simulink model "fuelsys_htmreq"  (Simulink 6.0)
settings: Solver=ode3  SolverMode=SingleTasking  StartTime=0.0  StopTime=2000  FixedStep=0.001  RelTol=1e-5  AbsTol=1e-6
PreLoadFcn:
  | load fsysdat
undefined symbols (not defined in the file): A1, A2, B1, B2, DISABLED, DiscIntNeverNeededParam, hys, Ki, LOW, max_ego, max_press, max_speed, max_throt, min_press, min_throt, o2_t_thresh, PressEst, pumpCon, RICH, SpeedEst, ThrotEst, zero_thresh
libraries: simulink x5, simulink_extras x3
settings Model: CovMetricSettings=dcmtr  Creator=The MathWorks Inc.  LastModifiedBy=batserve  ExtModeTrigMode=oneshot  ExtModeArmWhenConnect=off  ExtModeAutoUpdateStatusClock=off
settings DataIOCC: LimitDataPoints=off  SaveOutput=off  SaveTime=off  SignalLoggingName=logsOut
settings OptimizationCC: OptimizeModelRefInitCode=on  LifeSpan=1
settings DebuggingCC: CheckExecutionContextPreStartOutputMsg=on  CheckExecutionContextRuntimeOutputMsg=on  SolverPrmCheckMsg=none  IntegerOverflowMsg=none
settings ModelReferenceCC: UpdateModelReferenceTargets=IfOutOfDate
settings RTWCC: SystemTargetFile=ert.tlc  TemplateMakefile=ert_default_tmf  Description=RTW Embedded Coder (no auto configuration)  ProcessScript=ert_make_rtw_hook
settings ERTTargetCC: TargetFcnLib=ansi_tfl_tmw.mat  GenFloatMathFcnCalls=ANSI_C  GenerateSampleERTMain=on  SupportContinuousTime=on  SupportNonInlinedSFcns=on  RootIOFormat=Individual Arguments  ERTCustomFileTemplate=example_file_process.tlc  InitialValueSource=Model

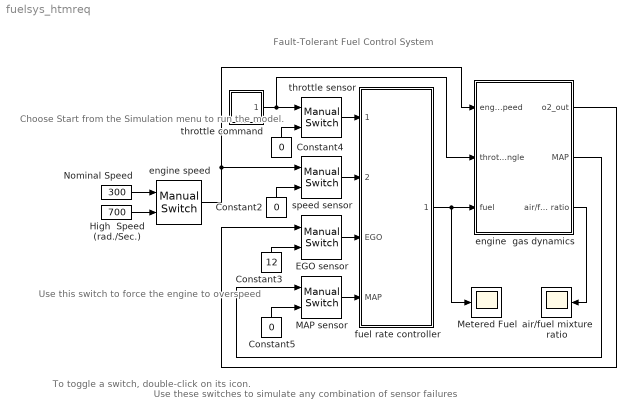
== system fuelsys_htmreq ==
  note: Use these switches to
      | simulate any combination
      | of sensor failures
  note: Use this switch
      | to force the
      | engine to
      | overspeed
  note: Fault-Tolerant Fuel Control System
  note: Choose Start from
      | the Simulation
      | menu to run
      | the model.
  note: To toggle
      | a switch,
      | double-click
      | on its icon.
  Constant2 : Constant  Orientation=up  Value=0
  Constant3 : Constant  Orientation=up  Value=12
  Constant4 : Constant  Orientation=up  Value=0
  Constant5 : Constant  Orientation=up  Value=0
  EGO sensor : simulink/Signal Routing/Manual Switch  sw=1  action=0
  High  Speed (rad./Sec.) : Constant  Value=700
  MAP sensor : simulink/Signal Routing/Manual Switch  sw=1  action=0
  Metered Fuel : Scope
      settings: TickLabels=on  TimeRange=8  YMin=0.75  YMax=2.25  DataFormat=Array
  Nominal Speed : Constant  Value=300
  air/fuel mixture ratio : Scope
      settings: TickLabels=on  TimeRange=8  YMin=11  YMax=16  DataFormat=Array
  engine speed : simulink/Signal Routing/Manual Switch  sw=1  action=0
  engine  gas dynamics : Subsystem  PropExecContextAcrossSSBoundary=on
  fuel rate controller : Subsystem  PropExecContextAcrossSSBoundary=on
  speed sensor : simulink/Signal Routing/Manual Switch  sw=1  action=0
  throttle command : Subsystem  PropExecContextAcrossSSBoundary=on  mask(Repeating table){rep_seq_t=[0 2 4], rep_seq_y=[10 20 10]}
      mask prompts: rep_seq_t "Time values:"; rep_seq_y "Output values:"
      mask help: Repeating table.
      mask init:
      | period = max(rep_seq_t);
      mask Help: Repeats cycle given in table. Time values should be monotonically increasing.
      mask Display: plot([rep_seq_t,rep_seq_t+period,rep_seq_t+2*period,rep_seq_t(1)+3*period],[rep_seq_y,rep_seq_y,rep_seq_y,rep_seq_y(1)])
  throttle sensor : simulink/Signal Routing/Manual Switch  sw=1  action=0
  wires:
  engine  gas dynamics/3(air/fuel ratio) -> air/fuel mixture ratio/1
  engine speed/1 -> engine  gas dynamics/1(engine speed), speed sensor/1
  MAP sensor/1 -> fuel rate controller/4(MAP)
  EGO sensor/1 -> fuel rate controller/3(EGO)
  speed sensor/1 -> fuel rate controller/2(engine speed)
  throttle sensor/1 -> fuel rate controller/1(throttle)
  fuel rate controller/1(fuel rate) -> engine  gas dynamics/3(fuel), Metered Fuel/1
  engine  gas dynamics/1(o2_out) -> EGO sensor/1
  Constant5/1 -> MAP sensor/2
  Constant3/1 -> EGO sensor/2
  throttle command/1(out_1) -> engine  gas dynamics/2(throttle angle), throttle sensor/1
  Constant2/1 -> speed sensor/2
  Constant4/1 -> throttle sensor/2
  engine  gas dynamics/2(MAP) -> MAP sensor/1
  High  Speed (rad./Sec.)/1 -> engine speed/2
  Nominal Speed/1 -> engine speed/1

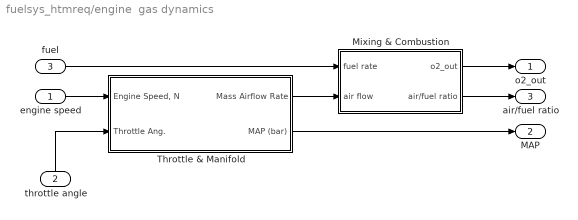
== system fuelsys_htmreq/engine  gas dynamics ==
  engine speed : Inport  Port=1  LatchInput=off
  throttle angle : Inport  Orientation=up  Port=2  LatchInput=off
  fuel : Inport  Port=3  LatchInput=off
  Mixing & Combustion : Subsystem  PropExecContextAcrossSSBoundary=on
  Throttle & Manifold : Subsystem  PropExecContextAcrossSSBoundary=on
  o2_out : Outport  InitialOutput=0
  MAP : Outport  Port=2  InitialOutput=0
  air/fuel ratio : Outport  Port=3  InitialOutput=0
  wires:
  Throttle & Manifold/1(Mass Airflow Rate) -> Mixing & Combustion/2(air flow)
  fuel/1 -> Mixing & Combustion/1(fuel rate)
  engine speed/1 -> Throttle & Manifold/1("Engine Speed, N")
  throttle angle/1 -> Throttle & Manifold/2(Throttle Ang.)
  Mixing & Combustion/2(air/fuel ratio) -> air/fuel ratio/1
  Throttle & Manifold/2(MAP (bar)) -> MAP/1
  Mixing & Combustion/1(o2_out) -> o2_out/1

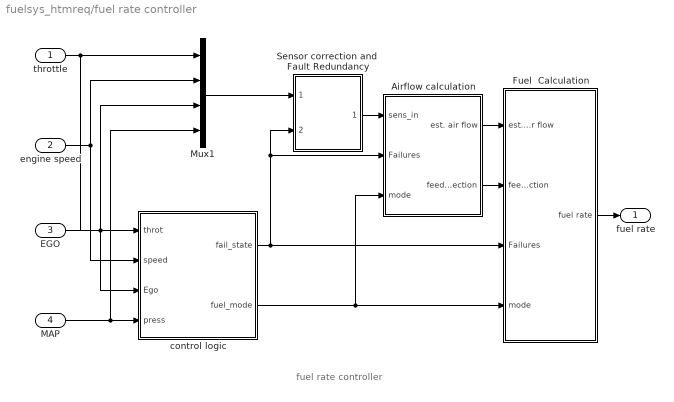
== system fuelsys_htmreq/fuel rate controller ==
  note: fuel rate controller
  throttle : Inport  Port=1  LatchInput=off
  engine speed : Inport  Port=2  LatchInput=off
  EGO : Inport  Port=3  LatchInput=off
  MAP : Inport  Port=4  LatchInput=off
  Airflow calculation : Subsystem  RequirementInfo={ 'HTML' 'fuelsys_requirements.htm' 'REQ1' 'true' 'Using a few parameters to estimate the mass airflow through the engine' 'REQ1' }  PropExecContextAcrossSSBoundary=on
  Fuel  Calculation : Subsystem  PropExecContextAcrossSSBoundary=on
  Mux1 : Mux
  Sensor correction and  Fault Redundancy : Subsystem  PropExecContextAcrossSSBoundary=on
  control logic : Stateflow chart  Description=Stateflow diagram to determine control system operating mode  PropExecContextAcrossSSBoundary=on
  fuel rate : Outport  InitialOutput=0
  wires:
  MAP/1 -> Mux1/4, control logic/4(press)
  EGO/1 -> Mux1/3, control logic/3(Ego)
  engine speed/1 -> Mux1/2, control logic/2(speed)
  throttle/1 -> Mux1/1, control logic/1(throt)
  Mux1/1 -> Sensor correction and  Fault Redundancy/1(Sensors)
  control logic/2(fuel_mode) -> Fuel  Calculation/4(mode), Airflow calculation/3(mode)
  Airflow calculation/2(feedback correction) -> Fuel  Calculation/2(feedback correction)
  Fuel  Calculation/1(fuel rate) -> fuel rate/1
  Airflow calculation/1(est. air flow) -> Fuel  Calculation/1(est. air flow)
  Sensor correction and  Fault Redundancy/1(Corrected) -> Airflow calculation/1(sens_in)
  control logic/1(fail_state) -> Sensor correction and  Fault Redundancy/2(Failures), Airflow calculation/2(Failures), Fuel  Calculation/3(Failures)

== system fuelsys_htmreq/throttle command ==
  Clock : Clock
      settings: Decimation=10
  Fcn1 : Fcn  Expr=rem(u[1],period)
  Look-Up Table : Lookup  DialogController=Simulink.DDGSource  InputValues=rep_seq_t  OutputValues=rep_seq_y  SaturateOnIntegerOverflow=on
  out_1 : Outport  InitialOutput=0
  wires:
  Look-Up Table/1 -> out_1/1
  Clock/1 -> Fcn1/1
  Fcn1/1 -> Look-Up Table/1

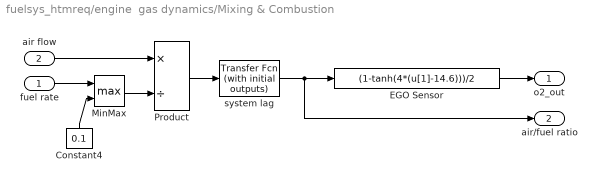
== system fuelsys_htmreq/engine  gas dynamics/Mixing & Combustion ==
  fuel rate : Inport  Port=1  LatchInput=off
  air flow : Inport  Port=2  LatchInput=off
  Constant4 : Constant  Orientation=up  Value=0.1
  EGO Sensor : Fcn  Expr=(1-tanh(4*(u[1]-14.6)))/2
  MinMax : MinMax  Function=max  Inputs=2  SaturateOnIntegerOverflow=on  InputSameDT=on
  Product : Product  Inputs=*/  SaturateOnIntegerOverflow=on  RndMeth=Zero  InputSameDT=on
  system lag : simulink_extras/Additional Linear/Transfer Fcn (with initial outputs)  N=3  D=[1 3]  Y0=1/14.6  U0=1/14.6
  o2_out : Outport  InitialOutput=0
  air/fuel ratio : Outport  Port=2  InitialOutput=0
  wires:
  Constant4/1 -> MinMax/2
  fuel rate/1 -> MinMax/1
  MinMax/1 -> Product/2
  Product/1 -> system lag/1
  system lag/1 -> air/fuel ratio/1, EGO Sensor/1
  EGO Sensor/1 -> o2_out/1
  air flow/1 -> Product/1

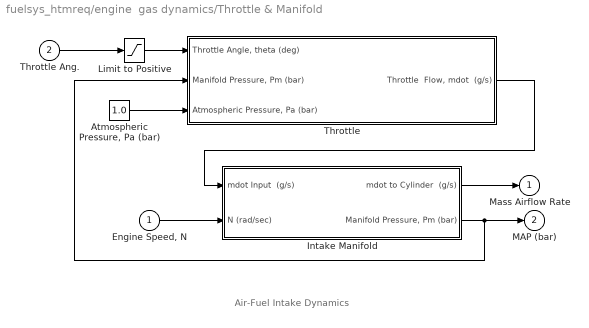
== system fuelsys_htmreq/engine  gas dynamics/Throttle & Manifold ==
  note: Air-Fuel Intake Dynamics
  "Engine Speed, N" : Inport  Port=1  LatchInput=off
  Throttle Ang. : Inport  Port=2  LatchInput=off
  "Atmospheric Pressure, Pa (bar)" : Constant  Value=1.0
  Intake Manifold : Subsystem  PropExecContextAcrossSSBoundary=on
  Limit to Positive : Saturate  UpperLimit=inf  LowerLimit=0
  Throttle : Subsystem  PropExecContextAcrossSSBoundary=on
  Mass Airflow Rate : Outport  InitialOutput=0
  MAP (bar) : Outport  Port=2  InitialOutput=0
  wires:
  Limit to Positive/1 -> Throttle/1("Throttle Angle, theta (deg)")
  Throttle Ang./1 -> Limit to Positive/1
  Throttle/1("Throttle  Flow, mdot  (g/s)") -> Intake Manifold/1(mdot Input  (g/s))
  "Engine Speed, N"/1 -> Intake Manifold/2(N (rad/sec))
  Intake Manifold/1(mdot to Cylinder  (g/s)) -> Mass Airflow Rate/1
  "Atmospheric Pressure, Pa (bar)"/1 -> Throttle/3("Atmospheric Pressure, Pa (bar) ")
  Intake Manifold/2("Manifold Pressure, Pm (bar)") -> Throttle/2("Manifold Pressure, Pm (bar)"), MAP (bar)/1

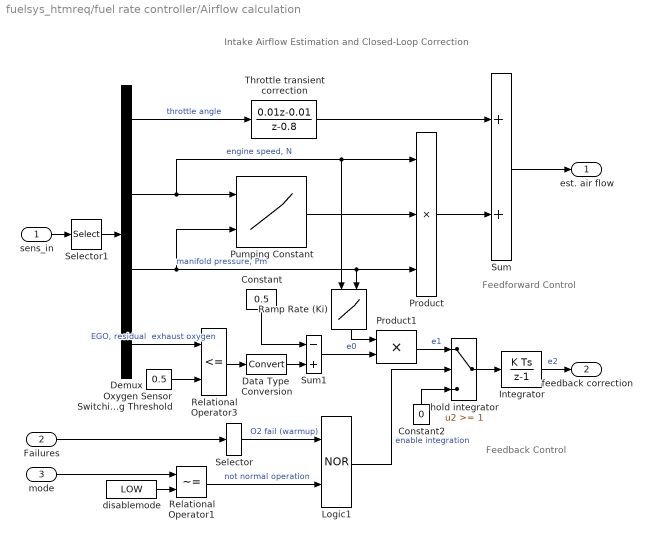
== system fuelsys_htmreq/fuel rate controller/Airflow calculation ==
  note: Intake Airflow Estimation and Closed-Loop Correction
  note: Feedback Control
  note: Feedforward Control
  sens_in : Inport  Port=1  LatchInput=off
  Failures : Inport  Port=2  LatchInput=off
  mode : Inport  Port=3  LatchInput=off
  Constant : Constant  Orientation=down  Value=0.5
  Constant2 : Constant  Orientation=up  Value=0
  Data Type  Conversion : DataTypeConversion  OutDataTypeMode=double  SaturateOnIntegerOverflow=on  RndMeth=Zero
  Demux : Demux
  Integrator : DiscreteIntegrator  RequirementInfo={ 'HTML' 'fuelsys_requirements.htm' 'REQ3' 'true' 'Use an exhaust sensor to adust the estimated airflow' 'REQ3' }  InitialCondition=-0.01  SampleTime=.01  ICPrevOutput=DiscIntNeverNeededParam  ICPrevScaledInput=DiscIntNeverNeededParam
  Logic1 : Logic  Operator=NOR
  Oxygen Sensor Switching Threshold : Constant  Value=0.5
  Product : Product  Inputs=3  SaturateOnIntegerOverflow=on  RndMeth=Zero  InputSameDT=on
  Product1 : Product  SaturateOnIntegerOverflow=on  RndMeth=Zero  InputSameDT=on
  Pumping Constant : Lookup2D  RequirementInfo={ 'HTML' 'fuelsys_requirements.htm' 'REQ2' 'true' 'Use a calibratible table to determine the pumping efficiency of the engine' 'REQ2' }  DialogController=Simulink.DDGSource  RowIndex=SpeedVect  ColumnIndex=press  OutputValues=pumpCon  SaturateOnIntegerOverflow=on  InputSameDT=on
  Ramp Rate (Ki) : Lookup2D  Orientation=down  DialogController=Simulink.DDGSource  RowIndex=[100:100:500]  ColumnIndex=[0:0.2:1]  OutputValues=[1:5]'*[1:6]*Ki  SaturateOnIntegerOverflow=on  InputSameDT=on
  Relational Operator1 : RelationalOperator  Operator=~=  InputSameDT=on
  Relational Operator3 : RelationalOperator  Operator=<=  InputSameDT=on
  Selector : Selector  Elements=3  InputPortWidth=4
  Selector1 : Selector  Elements=[1 2 4 3]  InputPortWidth=4
  Sum : Sum  Inputs=2  SaturateOnIntegerOverflow=on  InputSameDT=on
  Sum1 : Sum  Inputs=-+  SaturateOnIntegerOverflow=on  InputSameDT=on
  Throttle transient correction : DiscreteTransferFcn  Numerator=[0.01 -0.01]  Denominator=[1 -0.8]  SampleTime=.01
  disablemode : Constant  Value=LOW
  hold integrator : Switch  RequirementInfo={ 'HTML' 'fuelsys_requirements.htm' 'REQ6' 'true' 'Correction factor being held constant when oxygen sensor fails or in wamup mode' 'REQ6' }  Threshold=1  SaturateOnIntegerOverflow=on  InputSameDT=on
  est. air flow : Outport  InitialOutput=0
  feedback correction : Outport  Port=2  InitialOutput=0
  wires:
  Integrator/1 -> feedback correction/1  "e2"
  mode/1 -> Relational Operator1/1
  sens_in/1 -> Selector1/1
  Pumping Constant/1 -> Product/2
  Product/1 -> Sum/2
  Demux/3 -> Ramp Rate (Ki)/2, Product/3, Pumping Constant/2  "manifold pressure, Pm"
  Demux/2 -> Pumping Constant/1, Product/1, Ramp Rate (Ki)/1  "engine speed, N"
  Selector1/1 -> Demux/1
  Throttle transient correction/1 -> Sum/1
  Sum/1 -> est. air flow/1
  Demux/1 -> Throttle transient correction/1  "throttle angle"
  Selector/1 -> Logic1/1  "O2 fail (warmup)"
  Failures/1 -> Selector/1
  disablemode/1 -> Relational Operator1/2
  Relational Operator1/1 -> Logic1/2  "not normal operation"
  Demux/4 -> Relational Operator3/1  "EGO, residual  exhaust oxygen"
  Oxygen Sensor Switching Threshold/1 -> Relational Operator3/2
  Constant/1 -> Sum1/1
  Ramp Rate (Ki)/1 -> Product1/1
  Constant2/1 -> hold integrator/3
  Product1/1 -> hold integrator/1  "e1"
  hold integrator/1 -> Integrator/1
  Logic1/1 -> hold integrator/2  "enable integration"
  Sum1/1 -> Product1/2  "e0"
  Relational Operator3/1 -> Data Type  Conversion/1
  Data Type  Conversion/1 -> Sum1/2

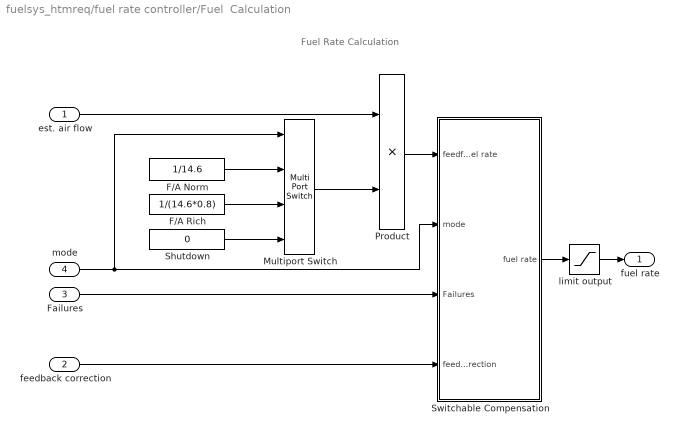
== system fuelsys_htmreq/fuel rate controller/Fuel  Calculation ==
  note: Fuel Rate Calculation
  est. air flow : Inport  Port=1  LatchInput=off
  feedback correction : Inport  Port=2  LatchInput=off
  Failures : Inport  Port=3  LatchInput=off
  mode : Inport  Port=4  LatchInput=off
  F/A Norm : Constant  Value=1/14.6
  F/A Rich : Constant  Value=1/(14.6*0.8)
  Multiport Switch : MultiPortSwitch  Inputs=3  SaturateOnIntegerOverflow=on  InputSameDT=on
  Product : Product  SaturateOnIntegerOverflow=on  RndMeth=Zero  InputSameDT=on
  Shutdown : Constant  Value=0
  Switchable Compensation : Subsystem  PropExecContextAcrossSSBoundary=on
  limit output : Saturate  UpperLimit=100  LowerLimit=0
  fuel rate : Outport  InitialOutput=0
  wires:
  limit output/1 -> fuel rate/1
  feedback correction/1 -> Switchable Compensation/4(feedback correction)
  Shutdown/1 -> Multiport Switch/4
  F/A Rich/1 -> Multiport Switch/3
  F/A Norm/1 -> Multiport Switch/2
  est. air flow/1 -> Product/1
  Multiport Switch/1 -> Product/2
  mode/1 -> Switchable Compensation/2(mode), Multiport Switch/1
  Failures/1 -> Switchable Compensation/3(Failures)
  Product/1 -> Switchable Compensation/1(feedforward fuel rate)
  Switchable Compensation/1(fuel rate) -> limit output/1

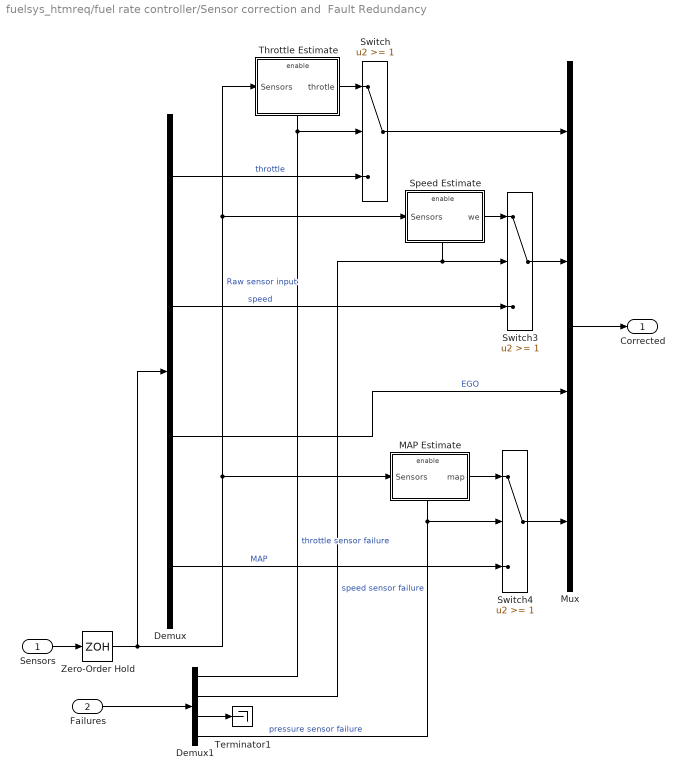
== system fuelsys_htmreq/fuel rate controller/Sensor correction and  Fault Redundancy ==
  Sensors : Inport  Port=1  LatchInput=off
  Failures : Inport  Port=2  LatchInput=off
  Demux : Demux
  Demux1 : Demux
  MAP Estimate : Subsystem  RequirementInfo={ 'HTML' 'fuelsys_requirements.htm' 'REQ8' 'true' 'When pressure sensor in failure mode, manifold pressure will be estimated' 'REG8' }  PropExecContextAcrossSSBoundary=on
  Mux : Mux
  Speed Estimate : Subsystem  PropExecContextAcrossSSBoundary=on
  Switch : Switch  Threshold=1  SaturateOnIntegerOverflow=on  InputSameDT=on
  Switch3 : Switch  Threshold=1  SaturateOnIntegerOverflow=on  InputSameDT=on
  Switch4 : Switch  Threshold=1  SaturateOnIntegerOverflow=on  InputSameDT=on
  Terminator1 : Terminator
  Throttle Estimate : Subsystem  PropExecContextAcrossSSBoundary=on
  Zero-Order Hold : ZeroOrderHold  SampleTime=0.01
  Corrected : Outport  InitialOutput=0
  wires:
  Sensors/1 -> Zero-Order Hold/1
  MAP Estimate/1(map) -> Switch4/1
  Demux/4 -> Switch4/3  "MAP"
  Switch4/1 -> Mux/4
  Demux1/4 -> Switch4/2, MAP Estimate/Enable  "pressure sensor failure"
  Demux1/2 -> Switch3/2, Speed Estimate/Enable  "speed sensor failure"
  Speed Estimate/1(we) -> Switch3/1
  Demux/2 -> Switch3/3  "speed"
  Switch3/1 -> Mux/2
  Demux1/1 -> Switch/2, Throttle Estimate/Enable  "throttle sensor failure"
  Demux1/3 -> Terminator1/1
  Throttle Estimate/1(throtle) -> Switch/1
  Demux/1 -> Switch/3  "throttle"
  Failures/1 -> Demux1/1
  Zero-Order Hold/1 -> Demux/1, Throttle Estimate/1(Sensors), Speed Estimate/1(Sensors), MAP Estimate/1(Sensors)  "Raw sensor input"
  Switch/1 -> Mux/1
  Demux/3 -> Mux/3  "EGO"
  Mux/1 -> Corrected/1

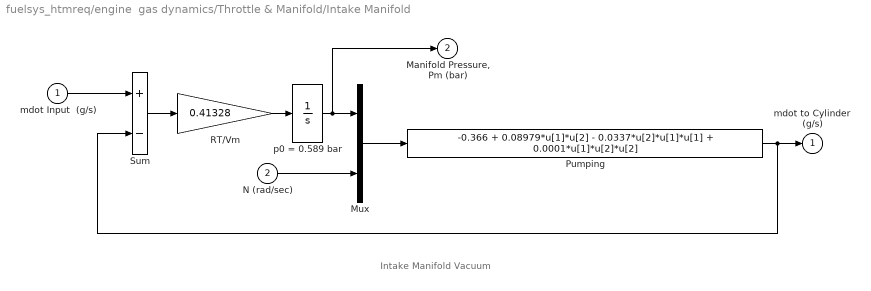
== system fuelsys_htmreq/engine  gas dynamics/Throttle & Manifold/Intake Manifold ==
  note: Intake Manifold Vacuum
  mdot Input  (g/s) : Inport  Port=1  LatchInput=off
  N (rad/sec) : Inport  Port=2  LatchInput=off
  Mux : Mux  Inputs=2
  Pumping : Fcn  Expr=-0.366 + 0.08979*u[1]*u[2] - 0.0337*u[2]*u[1]*u[1] + 0.0001*u[1]*u[2]*u[2]
  RT/Vm : Gain  Gain=0.41328  SaturateOnIntegerOverflow=on
  Sum : Sum  Inputs=+-  SaturateOnIntegerOverflow=on  InputSameDT=on
  p0 = 0.589 bar : Integrator  InitialCondition=.589
  mdot to Cylinder  (g/s) : Outport  InitialOutput=0
  "Manifold Pressure, Pm (bar)" : Outport  Port=2  InitialOutput=0
  wires:
  mdot Input  (g/s)/1 -> Sum/1
  RT/Vm/1 -> p0 = 0.589 bar/1
  N (rad/sec)/1 -> Mux/2
  Mux/1 -> Pumping/1
  p0 = 0.589 bar/1 -> Mux/1, "Manifold Pressure, Pm (bar)"/1
  Sum/1 -> RT/Vm/1
  Pumping/1 -> Sum/2, mdot to Cylinder  (g/s)/1

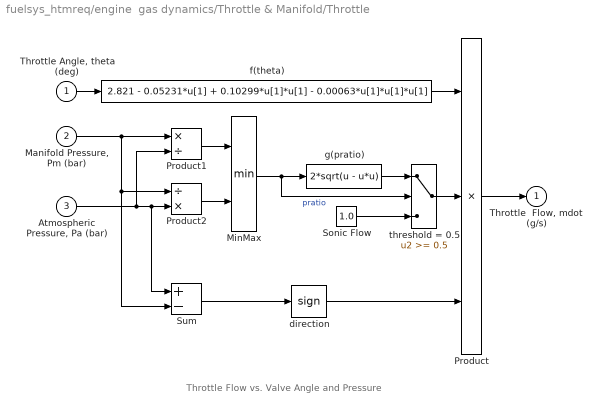
== system fuelsys_htmreq/engine  gas dynamics/Throttle & Manifold/Throttle ==
  note: Throttle Flow vs. Valve Angle and Pressure
  "Throttle Angle, theta (deg)" : Inport  Port=1  LatchInput=off
  "Manifold Pressure, Pm (bar)" : Inport  Port=2  LatchInput=off
  "Atmospheric Pressure, Pa (bar) " : Inport  Port=3  LatchInput=off
  MinMax : MinMax  Inputs=2  SaturateOnIntegerOverflow=on  InputSameDT=on
  Product : Product  Inputs=3  SaturateOnIntegerOverflow=on  RndMeth=Zero  InputSameDT=on
  Product1 : Product  Inputs=*/  SaturateOnIntegerOverflow=on  RndMeth=Zero  InputSameDT=on
  Product2 : Product  Inputs=/*  SaturateOnIntegerOverflow=on  RndMeth=Zero  InputSameDT=on
  "Sonic Flow " : Constant  Value=1.0
  Sum : Sum  Inputs=+-  SaturateOnIntegerOverflow=on  InputSameDT=on
  direction : Signum
  f(theta) : Fcn  Expr=2.821 - 0.05231*u[1] + 0.10299*u[1]*u[1] - 0.00063*u[1]*u[1]*u[1]
  g(pratio) : Fcn  Expr=2*sqrt(u - u*u)
  threshold = 0.5 : Switch  Threshold=0.5  SaturateOnIntegerOverflow=on  InputSameDT=on
  "Throttle  Flow, mdot  (g/s)" : Outport  InitialOutput=0
  wires:
  "Manifold Pressure, Pm (bar)"/1 -> Sum/2, Product2/1, Product1/1
  Product2/1 -> MinMax/2
  Product1/1 -> MinMax/1
  "Atmospheric Pressure, Pa (bar) "/1 -> Sum/1, Product2/2, Product1/2
  g(pratio)/1 -> threshold = 0.5/1
  "Sonic Flow "/1 -> threshold = 0.5/3
  threshold = 0.5/1 -> Product/2
  direction/1 -> Product/3
  Sum/1 -> direction/1
  MinMax/1 -> threshold = 0.5/2, g(pratio)/1  "pratio"
  "Throttle Angle, theta (deg)"/1 -> f(theta)/1
  Product/1 -> "Throttle  Flow, mdot  (g/s)"/1
  f(theta)/1 -> Product/1

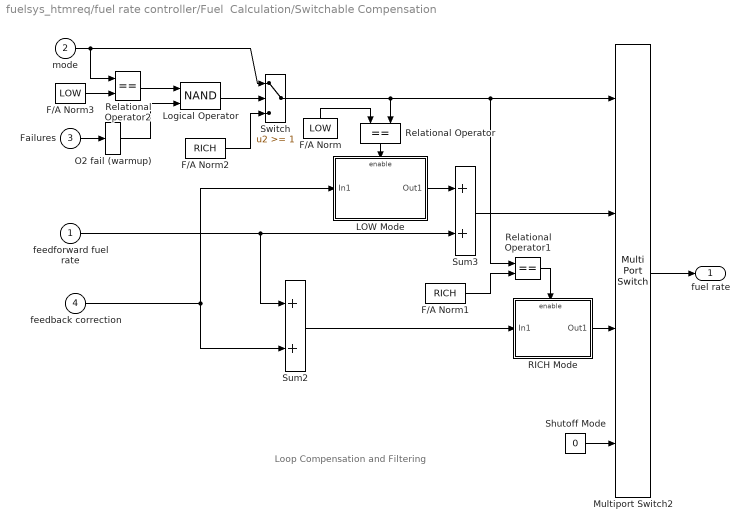
== system fuelsys_htmreq/fuel rate controller/Fuel  Calculation/Switchable Compensation ==
  note: Loop Compensation and Filtering
  feedforward fuel rate : Inport  Port=1  LatchInput=off
  mode : Inport  Port=2  LatchInput=off
  Failures : Inport  Port=3  LatchInput=off
  feedback correction : Inport  Port=4  LatchInput=off
  F/A Norm : Constant  Orientation=up  Value=LOW
  F/A Norm1 : Constant  Value=RICH
  F/A Norm2 : Constant  Value=RICH
  F/A Norm3 : Constant  Value=LOW
  LOW Mode : Subsystem  PropExecContextAcrossSSBoundary=on  mask(enabled discrete-time transfer function){num=B1, den=A1, u0=-0.01, y0=-0.01, Ts=0.01}
      mask prompts: num "numerator polynomial"; den "denominator polynomial"; u0 "initial input"; y0 "initial output"; Ts "sample time"
      mask Display: dpoly(num,den,'z')
  Logical Operator : Logic  Operator=NAND
  Multiport Switch2 : MultiPortSwitch  Inputs=3  SaturateOnIntegerOverflow=on  InputSameDT=on
  O2 fail (warmup) : Selector  Elements=3  InputPortWidth=4
  RICH Mode : Subsystem  PropExecContextAcrossSSBoundary=on  mask(enabled discrete-time transfer function){num=B2, den=A2, u0=1.6, y0=1.6, Ts=0.01}
      mask prompts: num "numerator polynomial"; den "denominator polynomial"; u0 "initial input"; y0 "initial output"; Ts "sample time"
      mask Display: dpoly(num,den,'z')
  Relational Operator : RelationalOperator  Orientation=down  Operator===  InputSameDT=on
  Relational Operator1 : RelationalOperator  Operator===  InputSameDT=on
  Relational Operator2 : RelationalOperator  Operator===  InputSameDT=on
  Shutoff Mode : Constant  Value=0
  Sum2 : Sum  SaturateOnIntegerOverflow=on  InputSameDT=on
  Sum3 : Sum  SaturateOnIntegerOverflow=on  InputSameDT=on
  Switch : Switch  Threshold=1  SaturateOnIntegerOverflow=on  InputSameDT=on
  fuel rate : Outport  InitialOutput=0
  wires:
  feedforward fuel rate/1 -> Sum3/2, Sum2/1
  feedback correction/1 -> LOW Mode/1(In1), Sum2/2
  RICH Mode/1(Out1) -> Multiport Switch2/3
  LOW Mode/1(Out1) -> Sum3/1
  Sum3/1 -> Multiport Switch2/2
  Sum2/1 -> RICH Mode/1(In1)
  Shutoff Mode/1 -> Multiport Switch2/4
  F/A Norm1/1 -> Relational Operator1/2
  Relational Operator1/1 -> RICH Mode/Enable
  Relational Operator/1 -> LOW Mode/Enable
  Multiport Switch2/1 -> fuel rate/1
  Switch/1 -> Relational Operator1/1, Multiport Switch2/1, Relational Operator/2
  F/A Norm/1 -> Relational Operator/1
  F/A Norm2/1 -> Switch/3
  Logical Operator/1 -> Switch/2
  mode/1 -> Switch/1, Relational Operator2/1
  F/A Norm3/1 -> Relational Operator2/2
  Relational Operator2/1 -> Logical Operator/1
  Failures/1 -> O2 fail (warmup)/1
  O2 fail (warmup)/1 -> Logical Operator/2

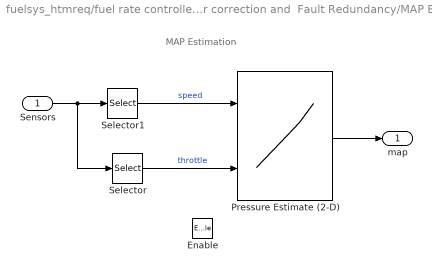
== system fuelsys_htmreq/fuel rate controller/Sensor correction and  Fault Redundancy/MAP Estimate ==
  note: MAP Estimation
  Sensors : Inport  Port=1  LatchInput=off
  Enable : EnablePort
  Pressure Estimate (2-D) : Lookup2D  DialogController=Simulink.DDGSource  RowIndex=SpeedVect  ColumnIndex=ThrotVect  OutputValues=PressEst  SaturateOnIntegerOverflow=on  InputSameDT=on
  Selector : Selector  InputPortWidth=4
  Selector1 : Selector  Elements=2  InputPortWidth=4
  map : Outport  InitialOutput=0
  wires:
  Sensors/1 -> Selector1/1, Selector/1
  Selector1/1 -> Pressure Estimate (2-D)/1  "speed"
  Selector/1 -> Pressure Estimate (2-D)/2  "throttle"
  Pressure Estimate (2-D)/1 -> map/1

== system fuelsys_htmreq/fuel rate controller/Sensor correction and  Fault Redundancy/Speed Estimate ==
  Sensors : Inport  Port=1  LatchInput=off
  Enable : EnablePort
  Selector : Selector  InputPortWidth=4
  Selector1 : Selector  Elements=4  InputPortWidth=4
  Speed Table (2-D) : Lookup2D  DialogController=Simulink.DDGSource  RowIndex=ThrotVect  ColumnIndex=press  OutputValues=SpeedEst  SaturateOnIntegerOverflow=on  InputSameDT=on
  we : Outport  InitialOutput=0
  wires:
  Speed Table (2-D)/1 -> we/1
  Sensors/1 -> Selector1/1, Selector/1
  Selector/1 -> Speed Table (2-D)/1  "throttle"
  Selector1/1 -> Speed Table (2-D)/2  "Manifold pressure"

== system fuelsys_htmreq/fuel rate controller/Sensor correction and  Fault Redundancy/Throttle Estimate ==
  Sensors : Inport  Port=1  LatchInput=off
  Enable : EnablePort
  Selector1 : Selector  Elements=4  InputPortWidth=4
  Selector2 : Selector  Elements=2  InputPortWidth=4
  Thrott Estimation Table (2-D) : Lookup2D  DialogController=Simulink.DDGSource  RowIndex=SpeedVect  ColumnIndex=press  OutputValues=ThrotEst  SaturateOnIntegerOverflow=on  InputSameDT=on
  throtle : Outport  InitialOutput=0
  wires:
  Sensors/1 -> Selector2/1, Selector1/1
  Selector2/1 -> Thrott Estimation Table (2-D)/1  "speed"
  Selector1/1 -> Thrott Estimation Table (2-D)/2  "Manifold pressure"
  Thrott Estimation Table (2-D)/1 -> throtle/1

== system fuelsys_htmreq/fuel rate controller/Fuel  Calculation/Switchable Compensation/LOW Mode ==
  In1 : Inport  Port=1  LatchInput=off
  Enable : EnablePort  StatesWhenEnabling=reset
  Discrete Transfer Fcn (with initial outputs) : simulink_extras/Additional Discrete/Discrete Transfer Fcn (with initial outputs)  N=num  D=den  U0=u0  Y0=y0  TS=Ts
  Out1 : Outport  InitialOutput=y0
  wires:
  Discrete Transfer Fcn (with initial outputs)/1 -> Out1/1
  In1/1 -> Discrete Transfer Fcn (with initial outputs)/1

== system fuelsys_htmreq/fuel rate controller/Fuel  Calculation/Switchable Compensation/RICH Mode ==
  In1 : Inport  Port=1  LatchInput=off
  Enable : EnablePort  StatesWhenEnabling=reset
  Discrete Transfer Fcn (with initial outputs) : simulink_extras/Additional Discrete/Discrete Transfer Fcn (with initial outputs)  N=num  D=den  U0=u0  Y0=y0  TS=Ts
  Out1 : Outport  InitialOutput=y0
  wires:
  In1/1 -> Discrete Transfer Fcn (with initial outputs)/1
  Discrete Transfer Fcn (with initial outputs)/1 -> Out1/1

== stateflow chart fuel rate controller/control logic ==
  settings: updateMethod=DISCRETE  sampleTime=0.01
  state Oxygen_Sensor_Mode [parallel]
    settings: description=This state determines the validity of the exhaust gas oxygen sensor (EGO) data.
    state O2_fail
      entry: fail_state[O2] = 1;
      settings: description=The EGO sensor has failed.
    state O2_warmup
      entry: fail_state[O2] = 1;
      settings: description=The EGO sensor must come up to temperature before its data is reliable.
    state O2_normal
      entry: fail_state[O2] = 0;
      settings: description=Normal EGO sensor operation gives a reliable indication of excess oxygen in the exhaust gas, from which air/fuel mixture can be inferred.
    O2_fail -> O2_normal : [Ego < max_ego] /
        | Sens_Failure_Counter.DEC
    O2_normal -> O2_fail : [Ego > max_ego]/
        | Sens_Failure_Counter.INC
      settings: description=The failure condition is indicated by excessive output voltage.
    (default) -> O2_warmup
    O2_warmup -> O2_normal : [t > o2_t_thresh]
      settings: description=It is assumed that the time o2_t_thresh is sufficient for the sensor to warm up to operational temperature.
  state Pressure_Sensor_Mode [parallel]
    settings: description=This state assesses the validity of the manifold absolute pressure (MAP) sensor.
    state press_norm
      entry:  fail_state[PRESS] = 0
      settings: description=The manifold pressure sensor gives a reliable indication of absolute pressure (MAP).
    state press_fail
      entry: fail_state[PRESS] = 1
      settings: description=The pressure sensor (manifold, or MAP) no longer produces reliable data.
    press_norm -> press_fail : [press > max_press | press < min_press]
        | /Sens_Failure_Counter.INC
    (default) -> press_norm
    press_fail -> press_norm : [press > min_press & press < max_press] /
        | Sens_Failure_Counter.DEC
  state Throttle_Sensor_Mode [parallel]
    settings: description=This state determines the validity of the throttle sensor signal.
    state throt_norm
      entry: fail_state[THROT] = 0;
      settings: description=The throttle sensor gives a reliable indication of the angle of the throttle plate.
    state throt_fail
      entry: fail_state[THROT] = 1;
      settings: description=Signal levels indicate that the throttle sensor data is no longer valid.
    throt_norm -> throt_fail : [throt> max_throt | throt < min_throt]/
        | Sens_Failure_Counter.INC
      settings: description=A failure is indicated by data which is outside the expected range, typically due to an open or short circuit.
    (default) -> throt_norm
    throt_fail -> throt_norm : [throt >  min_throt & throt < max_throt]
        | / Sens_Failure_Counter.DEC
  state Speed_Sensor_Mode [parallel]
    settings: description="This state infers the validity of the speed sensor data.  A failure is indicated by the presence of manifold vacuum at zero speed."
    state speed_norm
      entry: fail_state[SPEED] = 0
      settings: description=The speed sensor data accurately represents the engine speed.
    state speed_fail
      entry: fail_state[SPEED] = 1
      settings: description=The engine speed data is no longer available.
    speed_norm -> speed_fail : [speed==0 & press < zero_thresh]/
        | Sens_Failure_Counter.INC
      settings: description="Loss of a reliable speed sensor signal will indicate zero speed.  This is deemed invalid when the manifold vacuum indicates otherwise."
    (default) -> speed_norm
    speed_fail -> speed_norm : [speed > 0] /
        | Sens_Failure_Counter.DEC
  state Sens_Failure_Counter [parallel]
    settings: description=This state maintains a count of the number of sensors in failure mode.
    state MultiFail
      settings: description=This state represents any of the conditions in which more than one sensor is in failure mode.
      state FL3
        settings: description=Three of the engine sensors have failed.
      state FL4
        settings: description=All four of the engine sensors have failed.
      state FL2
        settings: description=Two of the engine sensors have failed.
      FL3 -> FL4 : INC
      FL2 -> FL3 : INC
      FL4 -> FL3 : DEC
      FL3 -> FL2 : DEC
    state FL1
      settings: description=One of the engine sensors has failed.
    state FL0
      settings: description=Zero failures; all sensors are operational.
    (default) -> FL0
    FL0 -> FL1 : INC
    FL1 -> FL2 : INC
    FL2 -> FL1 : DEC
    FL1 -> FL0 : DEC
  state Fueling_Mode [parallel]
    settings: description=This state interprets the other states in the chart to directly control the fueling mode.
    state Fuel_Disabled
      entry: fuel_mode = DISABLED
      settings: description=The fuel is completely shut off while in this state.
      state Overspeed
        settings: description=The speed is dangerously high, so shut off the fuel.
      state Shutdown
        settings: description=Cut off system operation due to multiple sensor failures.
      Overspeed -> (junction 35) : [in(speed_norm) & ...
          | speed < (max_speed - hys)]
      (junction 35) -> Shutdown : [in(MultiFail)]
    state Running
      settings: description=The fuel is actively controlled while in this state.
      (history)
      state Low_Emissions
        entry: fuel_mode = LOW
        (history)
        state Normal
          settings: description=All sensors are in correct operating modes, so effective closed-loop mixture control can be used.
        state Warmup
          settings: description="The sensors are all operational, but the oxygen (EGO) sensor is warming up.  We'll target a stoichiometric ratio, nonetheless, but won't close the loop around exhaust gas oxygen."
        (junction 36) -> Normal
        Warmup -> (junction 36) : [in(O2_normal)]
      state Rich_Mixture
        entry: fuel_mode = RICH
        settings: description=This mode enriches the mixture, lowering the air/fuel ratio.
        state Single_Failure
          settings: description=Continue uninterrupted engine operation, but with a richer mixture.
      Normal -> Single_Failure : [in(FL1)]
      Single_Failure -> Normal : [in(FL0)]
      (junction 36) -> Single_Failure : [in(FL1)]
    Running -> Overspeed : [ speed > max_speed ]
    (junction 35) -> Running : [!in(MultiFail)]
    Running -> Shutdown : enter(MultiFail)
    Shutdown -> Rich_Mixture : exit(MultiFail)
    (default) -> Warmup
  data: throt input double [0..120]; speed input double [0..1000]; Ego input double [0..12]; press input double [0..2]; fail_state output boolean size=4 [0..1]; fuel_mode output uint8 [1..3] =1; o2_t_thresh parameter double [0..60]; max_ego parameter double [0..2]; max_press parameter double [0..2]; min_press parameter double [0..2]; min_throt parameter double [0..120]; max_throt parameter double [0..120]; zero_thresh parameter double [0..450]; max_speed parameter double [0..1000]; hys parameter double [0..1000]; LOW parameter double; RICH parameter double; DISABLED parameter double; O2 constant uint8 =3; PRESS constant uint8 =4; THROT constant uint8 =1; SPEED constant uint8 =2
  data throt settings: units=degrees  description=throttle plate angle
  data speed settings: units=rad/sec  description=engine angular velocity
  data Ego settings: units=volts  description=Exhaust Gas Oxygen
  data press settings: units=bar (absolute)  description=Manifold Absolute Pressure (MAP)
  data fail_state settings: units=fail/ok  description=array of failure indications for use by Simulink model
  data fuel_mode settings: units=enumerated  description=fuel control mode: LOW = stoichiometric mixture, RICH = rich mixture, DISABLED = shut down
  data o2_t_thresh settings: units=sec  description=Time required to warm the EGO sensor sufficiently for valid data.
  data max_ego settings: units=volts  description=parameter represents the upper end of the EGO sensor range
  data max_press settings: units=bar (absolute)  description=parameter represents the upper limt of valid pressure readings
  data min_press settings: units=bar (absolute)  description=parameter for the lower end of the valid pressure sensor range
  data min_throt settings: units=degrees  description=minimum valid throttle angle
  data max_throt settings: units=degrees  description=parameter to indicate the maximum valid throttle angle reading
  data zero_thresh settings: units=bar (absolute)  description=minimum manifold pressure expected at zero speed
  data max_speed settings: units=rad/sec  description=parameter for the upper end of the safe engine speed range
  data hys settings: units=rad/sec  description=Hysteresis in the upper speed limit to avoid chatter at the threshold.
  data LOW settings: description="constant represents \"low emissions\" or stoichiometric fuel mixture mode"
  data RICH settings: description=constant represents rich fuel mixture mode
  data DISABLED settings: description=constant represents zero fuel mode
  data O2 settings: units=index  description=index into fail_state
  data PRESS settings: units=index  description=index into fail_state
  data THROT settings: units=index  description=index into fail_state
  data SPEED settings: units=index
  events: DEC local EITHER_EDGE_EVENT; INC local EITHER_EDGE_EVENT
